simulink model "mpc555rt_candbhost"  (Simulink 6.0)
settings: Solver=ode45  StartTime=0.0  StopTime=inf  RelTol=1e-3
libraries: vector_candrivers x4, canblocks x4
settings Model: Creator=The MathWorks Inc.  LastModifiedBy=batserve  ExtModeAutoUpdateStatusClock=off  ProdHWDeviceType=Specified
settings DataIOCC: SignalLoggingName=sigsOut
settings DebuggingCC: CheckExecutionContextPreStartOutputMsg=on  CheckExecutionContextRuntimeOutputMsg=on  SolverPrmCheckMsg=none
settings HardwareCC: ProdHWDeviceType=Specified

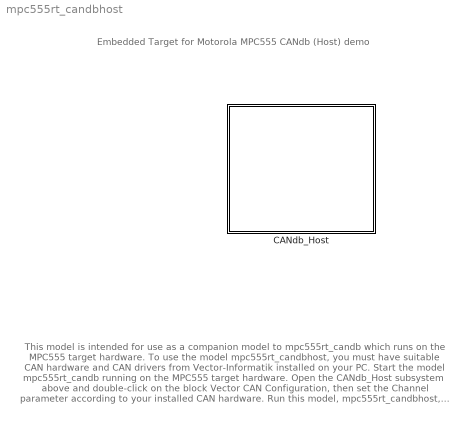
== system mpc555rt_candbhost ==
  note: This model is intended for use as a companion model to mpc555rt_candb which runs on the MPC555
      | target hardware. To use the model mpc555rt_candbhost, you must have suitable CAN hardware and
      | CAN drivers from Vector-Informatik installed on your PC.
      |
      | Start the model mpc555rt_candb running on the MPC555 target hardware.
      |
      | Open the CANdb_Host subsystem above and double-click on the block Vector CAN Configuration, then set
      | the Channel parameter according to your installed CAN hardware.
      |
      | Run this model, mpc555rt_candbhost, in Simulink on your host PC.
      |
      | CAN messages are sent between this model and the MPC555.   Unpacked messages are displayed in
      | the numeric display blocks, and on the scopes.   The messages transmitted by this model are
      | used to control MIOS Digital Outputs on the MPC555.
  note: Embedded Target for Motorola MPC555
      |                    CANdb (Host) demo
  CANdb_Host : Subsystem  PropExecContextAcrossSSBoundary=on

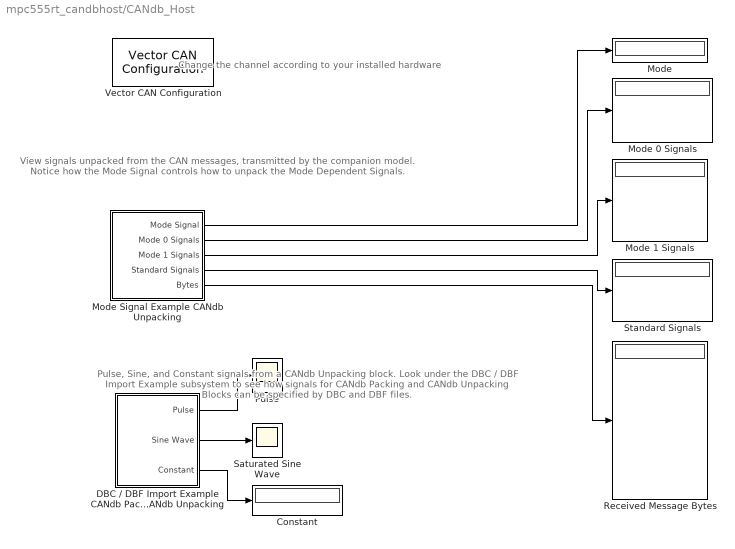
== system mpc555rt_candbhost/CANdb_Host ==
  note: Change the channel according
      | to your installed hardware
  note: View signals unpacked from the CAN messages,
      | transmitted by the companion model.
      | Notice how the Mode Signal controls how to unpack
      | the Mode Dependent Signals.
  note: Pulse, Sine, and Constant signals from
      | a CANdb Unpacking block.
      | Look under the DBC / DBF Import Example
      | subsystem to see how signals for CANdb
      | Packing and CANdb Unpacking Blocks
      | can be specified by DBC and DBF files.
  " Vector CAN Configuration  " : vector_candrivers/ Vector CAN Configuration  tag_param=config1  channel_param=None
  Constant : Display
  DBC / DBF Import Example CANdb Packing and CANdb Unpacking : Subsystem  PropExecContextAcrossSSBoundary=on
  Mode : Display
  Mode 0 Signals : Display
  Mode 1 Signals : Display
  Mode Signal Example CANdb Unpacking : Subsystem  PropExecContextAcrossSSBoundary=on
  Pulse : Scope
      settings: TimeRange=1000  YMin=0  YMax=1
  Received Message Bytes : Display
  Saturated Sine Wave : Scope
      settings: TimeRange=5000  YMin=-70  YMax=70
  Standard Signals : Display
  wires:
  Mode Signal Example CANdb Unpacking/1(Mode Signal) -> Mode/1
  Mode Signal Example CANdb Unpacking/4(Standard Signals) -> Standard Signals/1
  Mode Signal Example CANdb Unpacking/5(Bytes) -> Received Message Bytes/1
  Mode Signal Example CANdb Unpacking/2(Mode 0 Signals) -> Mode 0 Signals/1
  Mode Signal Example CANdb Unpacking/3(Mode 1 Signals) -> Mode 1 Signals/1
  DBC / DBF Import Example CANdb Packing and CANdb Unpacking/1(Pulse) -> Pulse/1
  DBC / DBF Import Example CANdb Packing and CANdb Unpacking/2(Sine Wave) -> Saturated Sine Wave/1
  DBC / DBF Import Example CANdb Packing and CANdb Unpacking/3(Constant) -> Constant/1

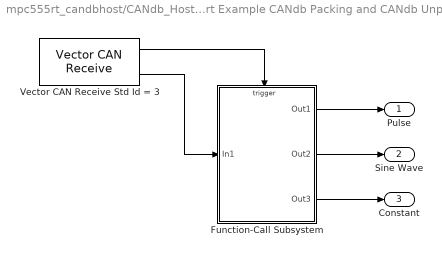
== system mpc555rt_candbhost/CANdb_Host/DBC / DBF Import Example CANdb Packing and CANdb Unpacking ==
  Function-Call Subsystem : Subsystem  TreatAsAtomicUnit=on  PropExecContextAcrossSSBoundary=on
  Vector CAN Receive Std Id = 3 : vector_candrivers/Vector CAN Receive  tag_param=config1  ids=3  frame_type_in=Standard (11-bit identifier)  sample_time=1  output_time=off  loop=on
  Pulse : Outport
  Sine Wave : Outport  Port=2
  Constant : Outport  Port=3
  wires:
  Function-Call Subsystem/3(Out3) -> Constant/1
  Function-Call Subsystem/2(Out2) -> Sine Wave/1
  Function-Call Subsystem/1(Out1) -> Pulse/1
  Vector CAN Receive Std Id = 3/2 -> Function-Call Subsystem/1(In1)
  Vector CAN Receive Std Id = 3/1 -> Function-Call Subsystem/Trigger

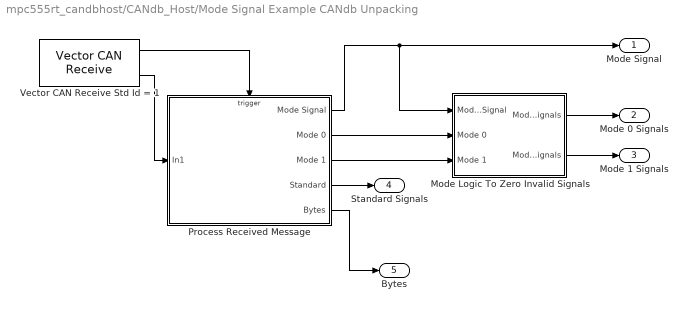
== system mpc555rt_candbhost/CANdb_Host/Mode Signal Example CANdb Unpacking ==
  Mode Logic To Zero Invalid Signals : Subsystem  PropExecContextAcrossSSBoundary=on
  Process Received Message : Subsystem  PropExecContextAcrossSSBoundary=on
  Vector CAN Receive Std Id = 1 : vector_candrivers/Vector CAN Receive  tag_param=config1  ids=1  frame_type_in=Standard (11-bit identifier)  sample_time=1  output_time=off  loop=on
  Mode Signal : Outport
  Mode 0 Signals : Outport  Port=2
  Mode 1 Signals : Outport  Port=3
  Standard Signals : Outport  Port=4
  Bytes : Outport  Port=5
  wires:
  Process Received Message/2(Mode 0) -> Mode Logic To Zero Invalid Signals/2(Mode 0)
  Mode Logic To Zero Invalid Signals/2(Mode 1 Signals) -> Mode 1 Signals/1
  Mode Logic To Zero Invalid Signals/1(Mode 0 Signals) -> Mode 0 Signals/1
  Process Received Message/5(Bytes) -> Bytes/1
  Process Received Message/4(Standard) -> Standard Signals/1
  Process Received Message/3(Mode 1) -> Mode Logic To Zero Invalid Signals/3(Mode 1)
  Process Received Message/1(Mode Signal) -> Mode Logic To Zero Invalid Signals/1(Mode Signal), Mode Signal/1
  Vector CAN Receive Std Id = 1/2 -> Process Received Message/1(In1)
  Vector CAN Receive Std Id = 1/1 -> Process Received Message/Trigger

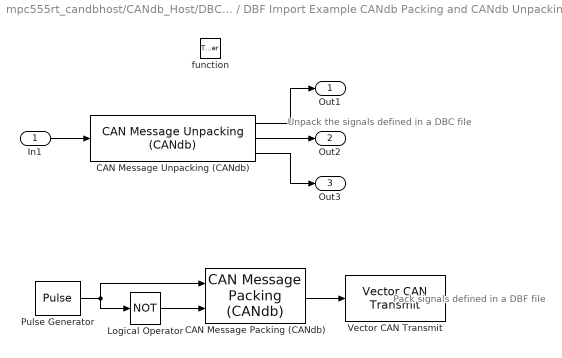
== system mpc555rt_candbhost/CANdb_Host/DBC / DBF Import Example CANdb Packing and CANdb Unpacking/Function-Call Subsystem ==
  note: Unpack the signals
      | defined in a DBC file
  note: Pack signals defined
      | in a DBF file
  In1 : Inport  Port=1  LatchInput=off
  function : TriggerPort  TriggerType=function-call
  CAN Message Packing (CANdb) : canblocks/CAN Message Packing (CANdb)
  CAN Message Unpacking (CANdb) : canblocks/CAN Message Unpacking (CANdb)/CAN Message Unpacking (CANdb)
  Logical Operator : Logic  Operator=NOT  AllPortsSameDT=off
  Pulse Generator : DiscretePulseGenerator  Period=20  PulseWidth=10  SampleTime=-1
  Vector CAN Transmit : vector_candrivers/Vector CAN Transmit  tag_param=config1  sample_time=-1
  Out1 : Outport
  Out2 : Outport  Port=2
  Out3 : Outport  Port=3
  wires:
  CAN Message Unpacking (CANdb)/3 -> Out3/1
  CAN Message Unpacking (CANdb)/2 -> Out2/1
  CAN Message Unpacking (CANdb)/1 -> Out1/1
  In1/1 -> CAN Message Unpacking (CANdb)/1
  CAN Message Packing (CANdb)/1 -> Vector CAN Transmit/1
  Pulse Generator/1 -> CAN Message Packing (CANdb)/1, Logical Operator/1
  Logical Operator/1 -> CAN Message Packing (CANdb)/2

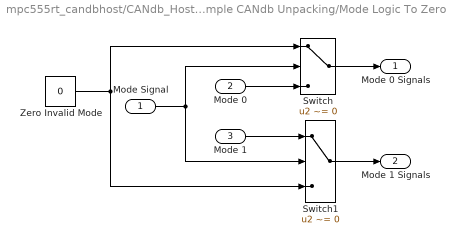
== system mpc555rt_candbhost/CANdb_Host/Mode Signal Example CANdb Unpacking/Mode Logic To Zero Invalid Signals ==
  Mode Signal : Inport  Port=1  LatchInput=off
  Mode 0 : Inport  Port=2  LatchInput=off
  Mode 1 : Inport  Port=3  LatchInput=off
  Switch : Switch  Criteria=u2 ~= 0  SaturateOnIntegerOverflow=on
  Switch1 : Switch  Criteria=u2 ~= 0  SaturateOnIntegerOverflow=on
  Zero Invalid Mode : Constant  Value=0
  Mode 0 Signals : Outport
  Mode 1 Signals : Outport  Port=2
  wires:
  Switch1/1 -> Mode 1 Signals/1
  Mode 1/1 -> Switch1/1
  Mode 0/1 -> Switch/3
  Switch/1 -> Mode 0 Signals/1
  Mode Signal/1 -> Switch/2, Switch1/2
  Zero Invalid Mode/1 -> Switch/1, Switch1/3

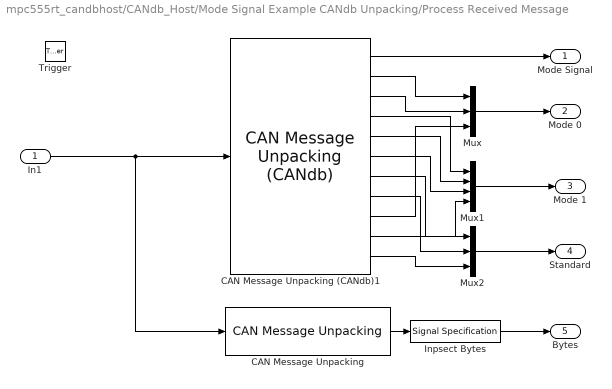
== system mpc555rt_candbhost/CANdb_Host/Mode Signal Example CANdb Unpacking/Process Received Message ==
  In1 : Inport  Port=1  LatchInput=off
  Trigger : TriggerPort  TriggerType=function-call
  CAN Message Unpacking : canblocks/CAN Message Unpacking/CAN Message Unpacking  showData=on  showID=off  showLength=off  endian=Little Endian (Intel)
  CAN Message Unpacking (CANdb)1 : canblocks/CAN Message Unpacking (CANdb)/CAN Message Unpacking (CANdb)
  Inpsect Bytes : SignalSpecification  Dimensions=8  DataType=uint8
  Mux : Mux  Inputs=3
  Mux1 : Mux
  Mux2 : Mux  Inputs=3
  Mode Signal : Outport
  Mode 0 : Outport  Port=2
  Mode 1 : Outport  Port=3
  Standard : Outport  Port=4
  Bytes : Outport  Port=5
  wires:
  Mux2/1 -> Standard/1
  CAN Message Unpacking (CANdb)1/11 -> Mux2/3
  CAN Message Unpacking (CANdb)1/8 -> Mux2/2
  CAN Message Unpacking (CANdb)1/7 -> Mux2/1
  Mux1/1 -> Mode 1/1
  CAN Message Unpacking (CANdb)1/10 -> Mux1/4
  CAN Message Unpacking (CANdb)1/6 -> Mux1/3
  CAN Message Unpacking (CANdb)1/5 -> Mux1/2
  CAN Message Unpacking (CANdb)1/4 -> Mux1/1
  Mux/1 -> Mode 0/1
  CAN Message Unpacking (CANdb)1/9 -> Mux/3
  CAN Message Unpacking (CANdb)1/3 -> Mux/2
  CAN Message Unpacking (CANdb)1/2 -> Mux/1
  CAN Message Unpacking (CANdb)1/1 -> Mode Signal/1
  Inpsect Bytes/1 -> Bytes/1
  CAN Message Unpacking/1 -> Inpsect Bytes/1
  In1/1 -> CAN Message Unpacking/1, CAN Message Unpacking (CANdb)1/1
